simulink model "Open_Loop_V_F_Control"  (R2021a)
settings: Solver=ode23  StartTime=0.0  StopTime=6  MaxStep=1e-6  MinStep=1e-7  RelTol=1e-5
model workspace (MAT data in the model file):
  P = 4
undefined symbols (not defined in the file): Vdc
libraries: spsIGBTDiodeLib x6, spsSeriesRLCBranchLib x3, spsAsynchronousMachineSIUnitsLib x1, simulink x1, eeStairGenerator x1, spsDCVoltageSourceLib x1, spspowerguiLib x1
settings Model: Creator=amank  LastModifiedBy=amank

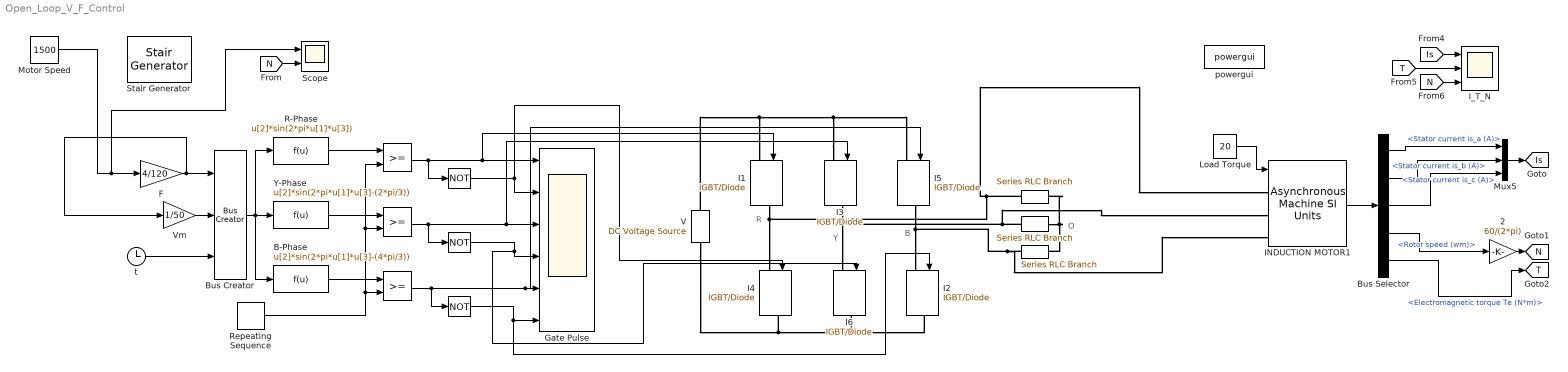
== system Open_Loop_V_F_Control ==
  note: Y
  note: O
  note: B
  note: R
  " " : RelationalOperator  OutDataTypeStr=boolean  RndMeth=Nearest
  "  " : RelationalOperator  OutDataTypeStr=boolean  RndMeth=Nearest
  "   " : RelationalOperator  OutDataTypeStr=boolean  RndMeth=Nearest
  "    " : Logic  Operator=NOT  AllPortsSameDT=off  OutDataTypeStr=boolean
  "     " : Logic  Operator=NOT  AllPortsSameDT=off  OutDataTypeStr=boolean
  "       " : Logic  Operator=NOT  AllPortsSameDT=off  OutDataTypeStr=boolean
  "          " : spsSeriesRLCBranchLib/Series RLC Branch  LConnTagsString=__new0  RConnTagsString=__new0  BranchType=R  Resistance=1  Inductance=10e-3  SetiL0=off  InitialCurrent=0  Capacitance=1e-6  Setx0=off  InitialVoltage=0  Measurements=None
  "             " : spsSeriesRLCBranchLib/Series RLC Branch  LConnTagsString=__new0  RConnTagsString=__new0  BranchType=R  Resistance=1  Inductance=10e-3  SetiL0=off  InitialCurrent=0  Capacitance=1e-6  Setx0=off  InitialVoltage=0  Measurements=None
  "                 " : spsSeriesRLCBranchLib/Series RLC Branch  LConnTagsString=__new0  RConnTagsString=__new0  BranchType=R  Resistance=1  Inductance=10e-3  SetiL0=off  InitialCurrent=0  Capacitance=1e-6  Setx0=off  InitialVoltage=0  Measurements=None
  " 2" : Gain  Gain=60/(2*pi)
  B-Phase : Fcn  Expr=u[2]*sin(2*pi*u[1]*u[3]-(4*pi/3))
  Bus Creator : BusCreator  Inputs=3
  Bus Selector : BusSelector  OutputSignals=Stator measurements.Stator current is_a (A),Stator measurements.Stator current is_b (A),Stator measurements.Stator current is_c (A),Mechanical.Rotor speed (wm),Mechanical.Electromagnetic torque Te (N*m)
  F : Gain  Gain=4/120
  Gate Pulse : Scope  NumInputPorts=6
  I{1..6} (6 alike) : spsIGBTDiodeLib/IGBT//Diode  Ron=1e-3  Rs=1e5  Cs=inf  Measurements=off
  INDUCTION MOTOR1 : spsAsynchronousMachineSIUnitsLib/Asynchronous Machine SI Units  RotorType=Squirrel-cage  PresetModel="15:  5.4 HP (4KW)   400 V  50Hz 1430 RPM"  MechanicalLoad=Torque Tm  ShowDetailedParameters=on  ReferenceFrame=Rotor  Units=SI  MeasurementBus=off  NominalParameters=[4000 400 50]  VoltageRatio=1  Stator=[1.405 0.005839]  Rotor=[1.395 0.005839]  Cage1=[ 0.022 0.226/377]  Cage2=[ 0.022 0.226/377]  Lm=0.1722  Mechanical=[0.0131 0.002985 2]  PolePairs=2  InitialConditions=[1 0 0 0 0 0 0 0]  SimulateSaturation=off  Saturation=[14.03593122, 27.81365428, 53.79336849, 72.68890987, 97.98006896, 148.6815601, 215.7428561, 302.9841135, 420.4778367 ; 230, 322, 414, 460, 506, 552, 598, 644, 690]  LoadFlowParameters=1492000  TsPowergui=0  TsBlock=-1  IterativeModel=Trapezoidal non iterative  IterativeDiscreteModel=Trapezoidal non iterative  Pmec=0
      settings: AttributesFormatString=\n
  I_T_N : Scope  NumInputPorts=3
  Load Torque : Constant  Value=20
  Motor Speed : Constant  Value=1500
  Mux5 : Mux  Inputs=3
  R-Phase : Fcn  Expr=u[2]*sin(2*pi*u[1]*u[3])
  Repeating Sequence : simulink/Sources/Repeating Sequence  rep_seq_t=[0 t/2 t]  rep_seq_y=[1 -1 1]
  Scope : Scope  NumInputPorts=2
  Stair Generator : eeStairGenerator/Stair Generator  LabelModeActiveChoice=Discrete  TimeInput=[0.0 2 4]  AmplitudeInput=[1000 1500 800]  SampleTime=1e-6  RepeatPattern=off  OutDataTypeStr=double
      settings: SourceProductBaseCode=PS
  V : spsDCVoltageSourceLib/DC Voltage Source  Amplitude=Vdc  Measurements=None
  Vm : Gain  Gain=1/50
  Y-Phase : Fcn  Expr=u[2]*sin(2*pi*u[1]*u[3]-(2*pi/3))
  powergui : spspowerguiLib/powergui  Priority=1  SimulationMode=Continuous  SampleTime=1e-6  frequency=60  Iterations=50  frequencyindice=0  Pbase=100e6  ErrMax=1e-4  UnitsV=kV  UnitsW=MW  buscounter=0  FunctionMessages=off  echomessages=off  EnableUseOfTLC=off  CurrentSourceSwitches=off  DisableSnubberDevices=off  DisableRonSwitches=off  DisableVfSwitches=off  DisplayEquations=off  AutomaticDiscreteSolvers=off  SolverType=Tustin/Backward Euler (TBE)  Interpol=off  ExternalGateDelay=off  methode=off  Ts=100  x0status=blocks  SPID=on  SwTol=0  HookPort=off  NonlinearTolerance=1e-4  nMaxIteration=100  ContinueOnMaxIteration=off  RestoreLinks=warning  ResistiveCurrentMeasurement=off  Frange=[0:2:500]  Ylog=off  Xlog=on  ShowGrid=off  save=off  variable=ZData  structure=VF_LO_V  ZoomFFT=off  StartTime=0.5  cycles=2  DisplayStyle=1  fundamental=50  FreqAxis=on  MaxFrequency=10000  frequencyindicesteady=1  RmsSteady=1  display=off
  t : Clock
  tag scope: Is=global, N=global, T=global
  wires:
  [T] -> I_T_N/2
  [Is] -> I_T_N/1
  [N] -> I_T_N/3
  R-Phase/1 -> " "/1
  Bus Creator/1 -> R-Phase/1, Y-Phase/1, B-Phase/1
  B-Phase/1 -> "   "/1
  t/1 -> Bus Creator/3
  Vm/1 -> Bus Creator/2
  F/1 -> Vm/1, Bus Creator/1
  Y-Phase/1 -> "  "/1
  Repeating Sequence/1 -> "   "/2, "  "/2, " "/2
  "     "/1 -> I6/1, Gate Pulse/4
  "  "/1 -> "     "/1, I3/1, Gate Pulse/3
  " "/1 -> "    "/1, I1/1, Gate Pulse/1
  "    "/1 -> Gate Pulse/2, I4/1
  "       "/1 -> I2/1, Gate Pulse/6
  "   "/1 -> "       "/1, I5/1, Gate Pulse/5
  INDUCTION MOTOR1/1 -> Bus Selector/1
  Mux5/1 -> [Is]
  " 2"/1 -> [N]
  Bus Selector/5 -> [T]  "<Electromagnetic torque Te (N*m)>"
  Bus Selector/1 -> Mux5/1  "<Stator current is_a (A)>"
  Load Torque/1 -> INDUCTION MOTOR1/1
  Bus Selector/4 -> " 2"/1  "<Rotor speed (wm)>"
  Bus Selector/2 -> Mux5/2  "<Stator current is_b (A)>"
  Bus Selector/3 -> Mux5/3  "<Stator current is_c (A)>"
  [N] -> Scope/2
  Motor Speed/1 -> Scope/1, F/1
  connections:
  "                 "/RConn1 -- "             "/RConn1 -- "          "/RConn1
  I3/LConn1 -- V/RConn1 -- I1/LConn1 -- I5/LConn1
  I4/RConn1 -- V/LConn1 -- I2/RConn1 -- I6/RConn1
  I3/RConn1 -- INDUCTION MOTOR1/LConn2 -- "          "/LConn1 -- I6/LConn1
  "             "/LConn1 -- I5/RConn1 -- I2/LConn1 -- INDUCTION MOTOR1/LConn3
  I1/RConn1 -- "                 "/LConn1 -- INDUCTION MOTOR1/LConn1 -- I4/LConn1
